simulink model "dinamics1"  (R2017a)
settings: Solver=VariableStepAuto  StartTime=0.0  StopTime=10  RelTol=1e-3
libraries: UR3_Lib x2, dspinverses x1
settings Model: Creator=dscat  LastModifiedBy=dscat

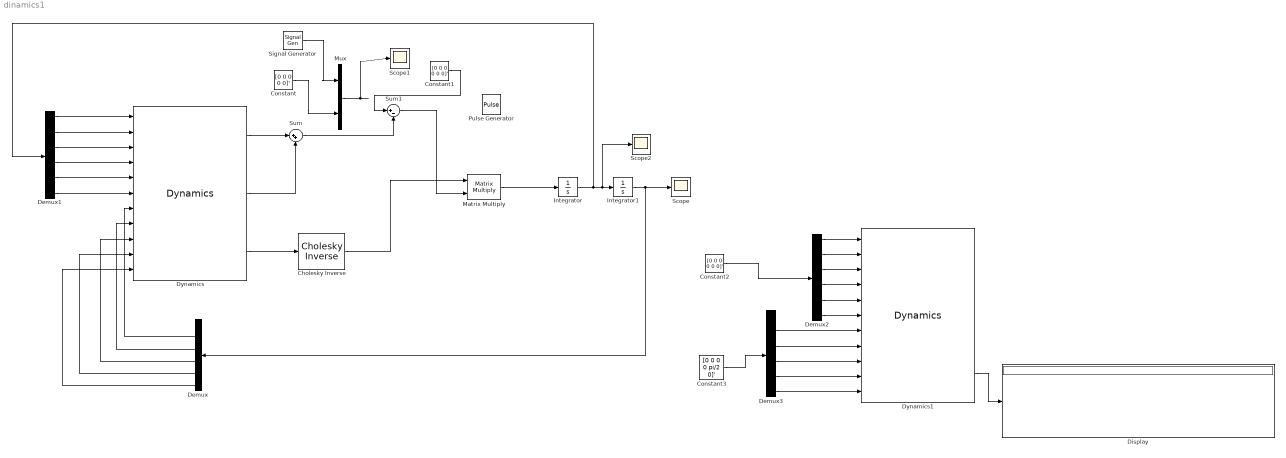
== system dinamics1 ==
  Cholesky Inverse : dspinverses/Cholesky Inverse  errmode=Warning
      settings: SourceProductName=DSP System Toolbox  SourceProductBaseCode=DS
  Constant : Constant  Value=[0 0 0 0 0]'
  Constant1 : Constant  Value=[0 0 0 0 0 0]'
  Constant2 : Constant  Value=[0 0 0 0 0 0]'
  Constant3 : Constant  Value=[0 0 0 0 pi/2 0]'
  Demux{,1..3} (4 alike) : Demux  Outputs=6
  Display : Display
  Dynamics : UR3_Lib/Dynamics
  Dynamics1 : UR3_Lib/Dynamics
  Integrator : Integrator  InitialCondition=[0 0 0 0 0 0]'
  Integrator1 : Integrator  InitialCondition=[0 0 0 0 0 0]'
  Matrix Multiply : Product  Multiplication=Matrix(*)
  Mux : Mux  Inputs=2
  Pulse Generator : DiscretePulseGenerator  PulseType=Time based  Amplitude=[1 0 0 0 0 0]  Period=3  PulseWidth=5
  Scope : Scope
  Scope1 : Scope
  Scope2 : Scope
  Signal Generator : SignalGenerator  WaveForm=square  Frequency=0.05
  Sum : Sum  Inputs=|++
  Sum1 : Sum  Inputs=|+-
  wires:
  Cholesky Inverse/1 -> Matrix Multiply/1
  Dynamics/2 -> Sum/2
  Dynamics/1 -> Sum/1
  Sum/1 -> Sum1/2
  Constant/1 -> Mux/2
  Sum1/1 -> Matrix Multiply/2
  Matrix Multiply/1 -> Integrator/1
  Integrator/1 -> Demux1/1, Scope2/1, Integrator1/1
  Integrator1/1 -> Demux/1, Scope/1
  Demux/2 -> Dynamics/7
  Demux/3 -> Dynamics/8
  Demux/4 -> Dynamics/9
  Demux/5 -> Dynamics/10
  Demux/6 -> Dynamics/11
  Demux1/6 -> Dynamics/6
  Demux1/5 -> Dynamics/5
  Demux1/4 -> Dynamics/4
  Demux1/3 -> Dynamics/3
  Demux1/2 -> Dynamics/2
  Demux1/1 -> Dynamics/1
  Mux/1 -> Scope1/1
  Signal Generator/1 -> Mux/1
  Constant1/1 -> Sum1/1
  Dynamics/3 -> Cholesky Inverse/1
  Constant3/1 -> Demux3/1
  Constant2/1 -> Demux2/1
  Demux2/1 -> Dynamics1/1
  Demux2/2 -> Dynamics1/2
  Demux2/3 -> Dynamics1/3
  Demux2/4 -> Dynamics1/4
  Demux2/5 -> Dynamics1/5
  Demux2/6 -> Dynamics1/6
  Demux3/6 -> Dynamics1/11
  Demux3/5 -> Dynamics1/10
  Demux3/4 -> Dynamics1/9
  Demux3/3 -> Dynamics1/8
  Demux3/2 -> Dynamics1/7
  Dynamics1/3 -> Display/1
